simulink model "springpend"  (R2021b)
settings: Solver=FixedStepAuto  StartTime=0.0  StopTime=100  FixedStep=0.01  RelTol=1e-3
settings Model: Creator=ПК  LastModifiedBy=ПК

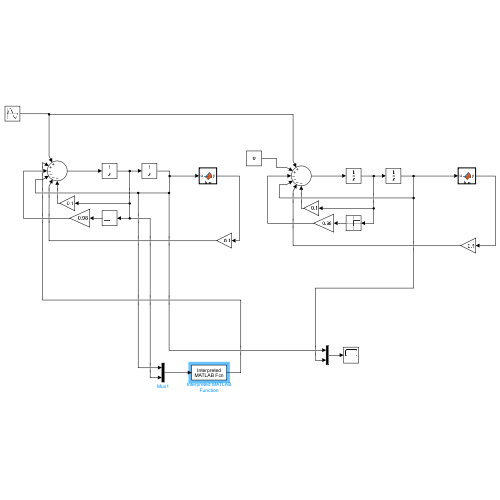
[thumbnail: Simulink's stored preview of the top-level diagram]
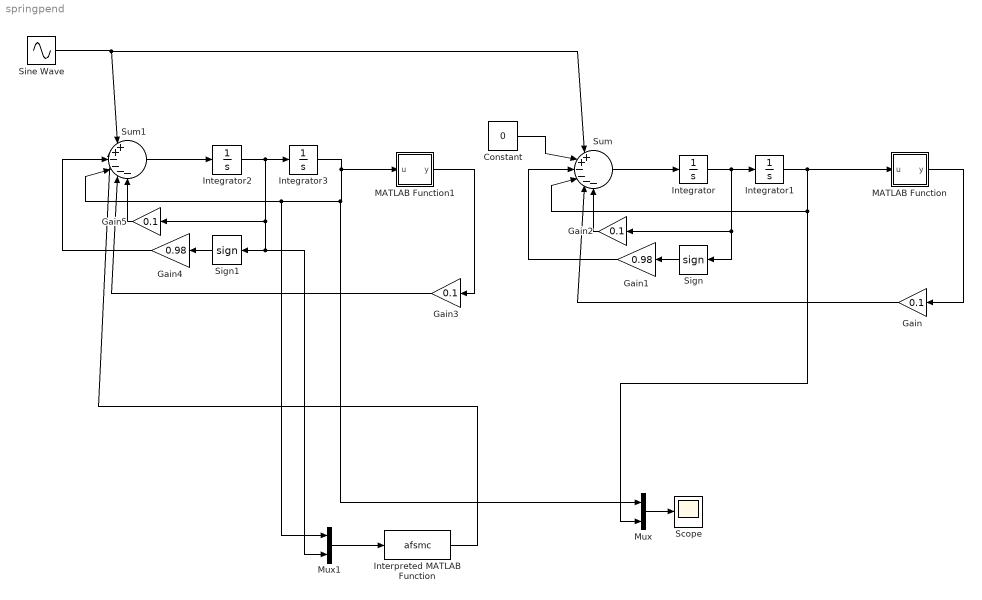
== system springpend ==
  Constant : Constant  Value=0
  Gain{,2..3,5} (4 alike) : Gain  Gain=0.1
  Gain1 : Gain  Gain=0.98
  Gain4 : Gain  Gain=0.98
  Integrator{,1..3} (4 alike) : Integrator
  Interpreted MATLAB Function : MATLABFcn  MATLABFcn=afsmc
  MATLAB Function : MATLAB Function  TreatAsAtomicUnit=on
  MATLAB Function1 : MATLAB Function  TreatAsAtomicUnit=on
  Mux : Mux  Inputs=2
  Mux1 : Mux  Inputs=2
  Scope : Scope
  Sign : Signum
  Sign1 : Signum
  Sine Wave : Sin  Amplitude=5  SampleTime=0
  Sum : Sum  Inputs=|++----
  Sum1 : Sum  Inputs=|++----
  wires:
  Sum/1 -> Integrator/1
  Integrator/1 -> Gain2/1, Sign/1, Integrator1/1
  Integrator1/1 -> MATLAB Function/1(u), Mux/2, Sum/4
  MATLAB Function/1(y) -> Gain/1
  Gain/1 -> Sum/5
  Sign/1 -> Gain1/1
  Gain1/1 -> Sum/3
  Gain2/1 -> Sum/6
  Constant/1 -> Sum/2
  Sum1/1 -> Integrator2/1
  Gain4/1 -> Sum1/3
  Integrator2/1 -> Gain5/1, Mux1/2, Sign1/1, Integrator3/1
  Gain3/1 -> Sum1/5
  Integrator3/1 -> MATLAB Function1/1(u), Mux/1, Mux1/1, Sum1/4
  Gain5/1 -> Sum1/6
  Sign1/1 -> Gain4/1
  MATLAB Function1/1(y) -> Gain3/1
  Mux/1 -> Scope/1
  Sine Wave/1 -> Sum/1, Sum1/1
  Mux1/1 -> Interpreted MATLAB Function/1
  Interpreted MATLAB Function/1 -> Sum1/2

== matlab function springpend/MATLAB Function ==
  data: u input; y output
function y = fcn(u)

y = u^3;

== matlab function springpend/MATLAB Function1 ==
  data: u input; y output
function y = fcn(u)

y = u^3;
